simulink model "modelofisicocompleto"  (R2017a)
settings: Solver=VariableStepAuto  StartTime=0.0  StopTime=20  MaxStep=1e-5  RelTol=1e-5
values from neighbouring files (symbols this model uses):
  bcx = 1000    [datoscarro.m]
  bcy = 500    [datoscarro.m]
  Beqtran = (0 + Beqrot/(Rr^2))    (= 27000)    [datoscarro.m]
  Bheqd = (bh  + (beqd/(Rd^2)))    (= 32)    [datoscarro.m]
  bw = 30000    [datoscarro.m]
  g = 9.82    [datoscarro.m]
  Kcy = 1.3e6    (= 1300000)    [datoscarro.m]
  Kw = 1800000    [datoscarro.m]
  lh0 = 10    [datoscarro.m]
  Meq = (mc + Jeq/(Rr^2))    (= 59008)    [datoscarro.m]
  Mheq = (Mh + (Jeqd/(Rd^2)))    (= 48014.2222222)    [datoscarro.m]
  Rd = 0.75    [datoscarro.m]
  Rr = 0.5    [datoscarro.m]
  rt = 15.0    (= 15)    [datoscarro.m]
  rtd = 30    [datoscarro.m]
  xl0 = 5    [datoscarro.m]
  xt0 = xl0    (= 5)    [datoscarro.m]    (also in plot_scene.m = -20)
  yl0 = yt0 - l0    (= 34.9181666667)    [datoscarro.m]
  yt0 = 45    [datoscarro.m]
settings Model: Creator=tomas  LastModifiedBy=tomas

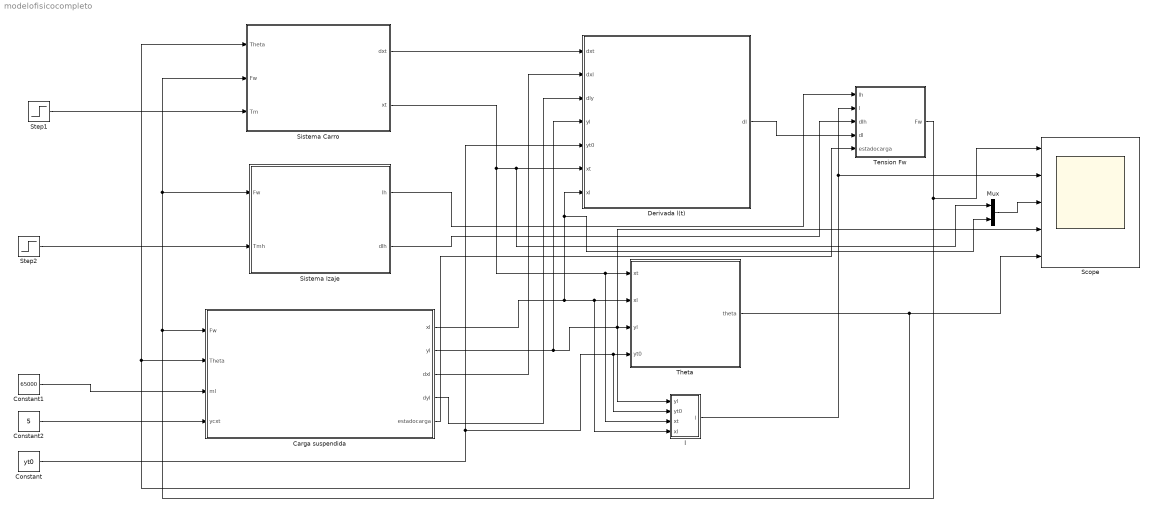
== system modelofisicocompleto ==
  Carga suspendida : Subsystem
  Constant : Constant  Value=yt0
  Constant1 : Constant  Value=65000
  Constant2 : Constant  Value=5
  Derivada l(t) : Subsystem
  Mux : Mux  Inputs=2
  Scope : Scope  NumInputPorts=5
  Sistema Carro : Subsystem
  Sistema Izaje : Subsystem
  Step1 : Step  Time=0  After=1000  SampleTime=0
  Step2 : Step  Time=0  After=25000  SampleTime=0
  Tension Fw : Subsystem
  Theta : Subsystem
  l : Subsystem
  wires:
  Step1/1 -> Sistema Carro/3(Tm)
  Sistema Carro/2(xt) -> l/3(xt), Theta/1(xt), Mux/1, Derivada l(t)/6(xt)
  Sistema Carro/1("dxt ") -> Derivada l(t)/1(dxt)
  Sistema Izaje/1(lh) -> Tension Fw/1(lh)
  Sistema Izaje/2(dlh) -> Tension Fw/3(dlh)
  Carga suspendida/1(xl) -> Mux/2, Derivada l(t)/7(xl), l/4(xl), Theta/2(xl)
  Carga suspendida/2(yl) -> l/1(yl), Theta/3(yl), Scope/4, Derivada l(t)/4(yl)
  Carga suspendida/3(dxl) -> Derivada l(t)/2(dxl)
  Carga suspendida/4(dyl) -> Derivada l(t)/3(dly)
  Derivada l(t)/1(dl) -> Tension Fw/4(dl)
  Constant/1 -> l/2(yt0), Theta/4(yt0), Derivada l(t)/5(yt0)
  l/1("l ") -> Scope/2, Tension Fw/2(l)
  Tension Fw/1("Fw ") -> Sistema Carro/2(Fw), Sistema Izaje/1(Fw), Carga suspendida/1(Fw), Scope/1
  Constant1/1 -> Carga suspendida/3(ml)
  Constant2/1 -> Carga suspendida/4(ycxt)
  Carga suspendida/5("estadocarga ") -> Tension Fw/5(estadocarga)
  Mux/1 -> Scope/3
  Step2/1 -> Sistema Izaje/2(Tmh)
  Theta/1("theta ") -> Scope/5, Sistema Carro/1(Theta), Carga suspendida/2(Theta)

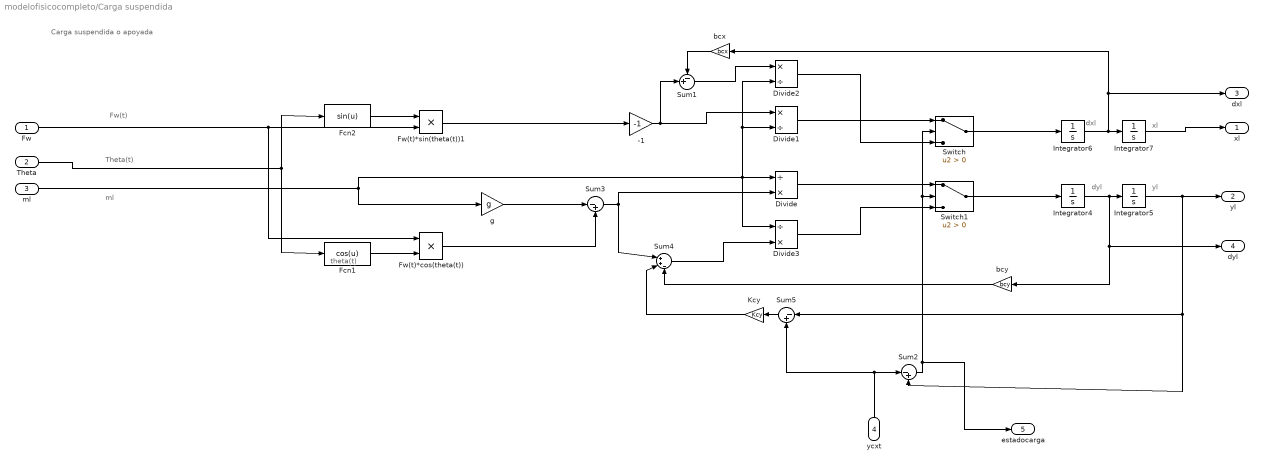
== system modelofisicocompleto/Carga suspendida ==
  note: Carga suspendida o apoyada
  note: Theta(t)
  note: Fw(t)
  note: ml
  note: theta(t)
  note: dyl
  note: yl
  note: dxl
  note: xl
  Fw : Inport
  Theta : Inport  Port=2
  ml : Inport  Port=3
  ycxt : Inport  Port=4
  -1 : Gain  Gain=-1
  Divide : Product  Inputs=/*
  Divide1 : Product  Inputs=*/
  Divide2 : Product  Inputs=*/
  Divide3 : Product  Inputs=/*
  Fcn1 : Fcn  Expr=cos(u)
  Fcn2 : Fcn  Expr=sin(u)
  Fw(t)*cos(theta(t)) : Product
  Fw(t)*sin(theta(t))1 : Product
  Integrator4 : Integrator
  Integrator5 : Integrator  InitialCondition=yl0
  Integrator6 : Integrator
  Integrator7 : Integrator  InitialCondition=xl0
  Kcy : Gain  Gain=Kcy
  Sum1 : Sum  Inputs=-+|
  Sum2 : Sum  Inputs=|-+
  Sum3 : Sum  Inputs=|-+
  Sum4 : Sum  Inputs=|++-
  Sum5 : Sum  Inputs=|-+
  Switch : Switch  Criteria=u2 > Threshold
  Switch1 : Switch  Criteria=u2 > Threshold
  bcx : Gain  Gain=bcx
  bcy : Gain  Gain=bcy
  g : Gain  Gain=g
  xl : Outport
  yl : Outport  Port=2
  dxl : Outport  Port=3
  dyl : Outport  Port=4
  "estadocarga " : Outport  Port=5
  wires:
  Fcn2/1 -> Fw(t)*sin(theta(t))1/1
  Theta/1 -> Fcn1/1, Fcn2/1
  g/1 -> Sum3/1
  Fcn1/1 -> Fw(t)*cos(theta(t))/2
  Fw(t)*cos(theta(t))/1 -> Sum3/2
  Fw/1 -> Fw(t)*cos(theta(t))/1, Fw(t)*sin(theta(t))1/2
  ml/1 -> g/1, Divide1/2, Divide2/2, Divide3/1, Divide/1
  Integrator7/1 -> xl/1
  Integrator6/1 -> bcx/1, dxl/1, Integrator7/1
  Fw(t)*sin(theta(t))1/1 -> -1/1
  Integrator5/1 -> Sum2/2, Sum5/1, yl/1
  Divide1/1 -> Switch/1
  -1/1 -> Sum1/2, Divide1/1
  Integrator4/1 -> dyl/1, bcy/1, Integrator5/1
  Sum3/1 -> Sum4/1, Divide/2
  Switch/1 -> Integrator6/1
  bcx/1 -> Sum1/1
  Sum2/1 -> "estadocarga "/1, Switch1/2, Switch/2
  ycxt/1 -> Sum2/1, Sum5/2
  Sum1/1 -> Divide2/1
  Divide2/1 -> Switch/3
  Sum4/1 -> Divide3/2
  Divide3/1 -> Switch1/3
  Switch1/1 -> Integrator4/1
  Divide/1 -> Switch1/1
  Sum5/1 -> Kcy/1
  Kcy/1 -> Sum4/2
  bcy/1 -> Sum4/3

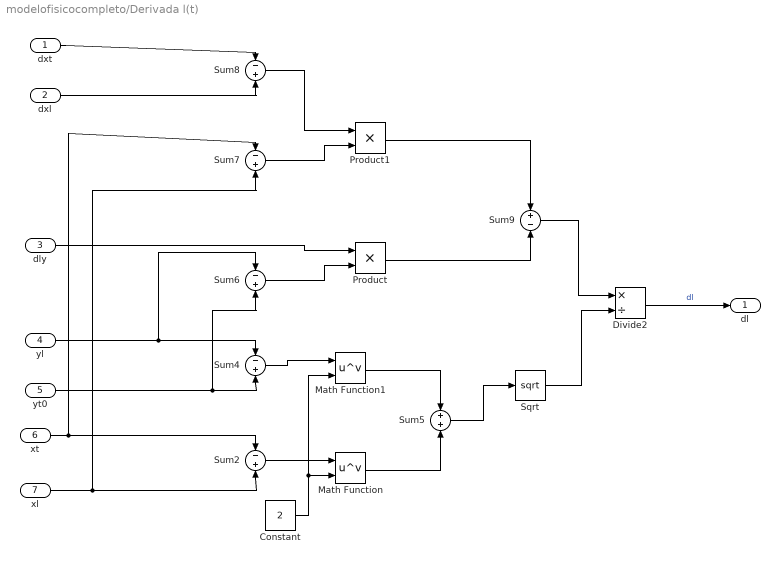
== system modelofisicocompleto/Derivada l(t) ==
  dxt : Inport
  dxl : Inport  Port=2
  dly : Inport  Port=3
  yl : Inport  Port=4
  yt0 : Inport  Port=5
  xt : Inport  Port=6
  xl : Inport  Port=7
  Constant : Constant  Value=2
  Divide2 : Product  Inputs=*/
  Math Function : Math  Operator=pow  SaturateOnIntegerOverflow=on
  Math Function1 : Math  Operator=pow  SaturateOnIntegerOverflow=on
  Product : Product
  Product1 : Product
  Sqrt : Sqrt  SaturateOnIntegerOverflow=on
  Sum{2,4,6..8} (5 alike) : Sum  Inputs=-+
  Sum5 : Sum
  Sum9 : Sum  Inputs=+-
  dl : Outport
  wires:
  Divide2/1 -> dl/1  "dl"
  dly/1 -> Product/1
  yl/1 -> Sum6/1, Sum4/1
  xl/1 -> Sum7/2, Sum2/2
  Product/1 -> Sum9/2
  dxt/1 -> Sum8/1
  Sum5/1 -> Sqrt/1
  Constant/1 -> Math Function1/2, Math Function/2
  yt0/1 -> Sum4/2, Sum6/2
  dxl/1 -> Sum8/2
  Math Function1/1 -> Sum5/1
  Sum8/1 -> Product1/1
  Sum9/1 -> Divide2/1
  Math Function/1 -> Sum5/2
  xt/1 -> Sum7/1, Sum2/1
  Sum6/1 -> Product/2
  Sum7/1 -> Product1/2
  Product1/1 -> Sum9/1
  Sum4/1 -> Math Function1/1
  Sqrt/1 -> Divide2/2
  Sum2/1 -> Math Function/1

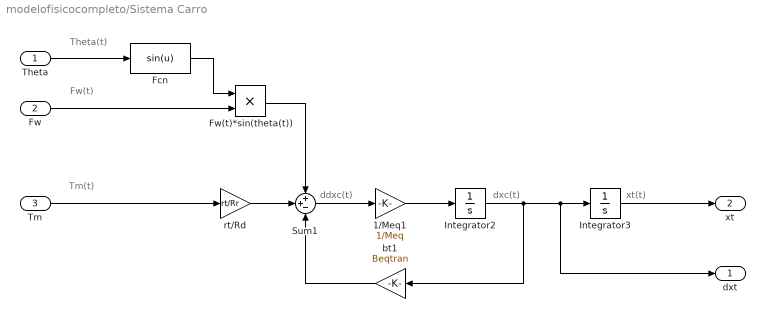
== system modelofisicocompleto/Sistema Carro ==
  note: dxc(t)
  note: xt(t)
  note: ddxc(t)
  note: Theta(t)
  note: Fw(t)
  note: Tm(t)
  Theta : Inport
  Fw : Inport  Port=2
  Tm : Inport  Port=3
  1/Meq1 : Gain  Gain=1/Meq
  Fcn : Fcn  Expr=sin(u)
  Fw(t)*sin(theta(t)) : Product
  Integrator2 : Integrator
  Integrator3 : Integrator  InitialCondition=xt0
  Sum1 : Sum  Inputs=++-
  bt1 : Gain  Gain=Beqtran
  rt/Rd : Gain  Gain=rt/Rr
  "dxt " : Outport
  xt : Outport  Port=2
  wires:
  Integrator3/1 -> xt/1
  Sum1/1 -> 1/Meq1/1
  Fw/1 -> Fw(t)*sin(theta(t))/2
  Fcn/1 -> Fw(t)*sin(theta(t))/1
  rt/Rd/1 -> Sum1/2
  Theta/1 -> Fcn/1
  Fw(t)*sin(theta(t))/1 -> Sum1/1
  1/Meq1/1 -> Integrator2/1
  Tm/1 -> rt/Rd/1
  bt1/1 -> Sum1/3
  Integrator2/1 -> bt1/1, "dxt "/1, Integrator3/1

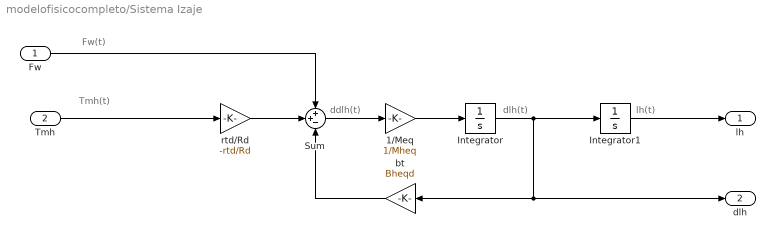
== system modelofisicocompleto/Sistema Izaje ==
  note: lh(t)
  note: dlh(t)
  note: ddlh(t)
  note: Tmh(t)
  note: Fw(t)
  Fw : Inport
  Tmh : Inport  Port=2
  1/Meq : Gain  Gain=1/Mheq
  Integrator : Integrator
  Integrator1 : Integrator  InitialCondition=lh0
  Sum : Sum  Inputs=++-
  bt : Gain  Gain=Bheqd
  rtd/Rd : Gain  Gain=-rtd/Rd
  lh : Outport
  dlh : Outport  Port=2
  wires:
  Integrator/1 -> dlh/1, bt/1, Integrator1/1
  Integrator1/1 -> lh/1
  rtd/Rd/1 -> Sum/2
  bt/1 -> Sum/3
  Fw/1 -> Sum/1
  Tmh/1 -> rtd/Rd/1
  1/Meq/1 -> Integrator/1
  Sum/1 -> 1/Meq/1

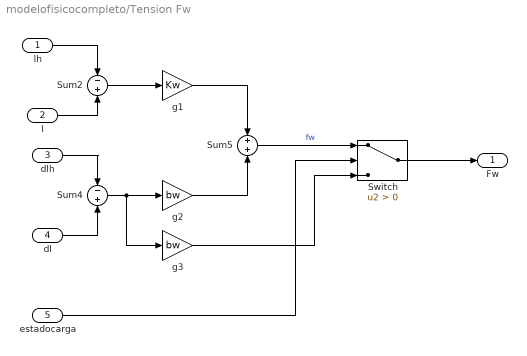
== system modelofisicocompleto/Tension Fw ==
  lh : Inport
  l : Inport  Port=2
  dlh : Inport  Port=3
  dl : Inport  Port=4
  estadocarga : Inport  Port=5
  Sum2 : Sum  Inputs=-+
  Sum4 : Sum  Inputs=-+
  Sum5 : Sum
  Switch : Switch  Criteria=u2 > Threshold
  g1 : Gain  Gain=Kw
  g2 : Gain  Gain=bw
  g3 : Gain  Gain=bw
  "Fw " : Outport
  wires:
  l/1 -> Sum2/2
  lh/1 -> Sum2/1
  dl/1 -> Sum4/2
  g2/1 -> Sum5/2
  Sum5/1 -> Switch/1  "fw"
  Sum4/1 -> g3/1, g2/1
  g1/1 -> Sum5/1
  dlh/1 -> Sum4/1
  Sum2/1 -> g1/1
  Switch/1 -> "Fw "/1
  estadocarga/1 -> Switch/2
  g3/1 -> Switch/3

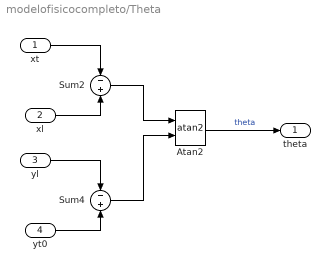
== system modelofisicocompleto/Theta ==
  xt : Inport
  xl : Inport  Port=2
  yl : Inport  Port=3
  yt0 : Inport  Port=4
  Atan2 : Trigonometry  Operator=atan2
  Sum2 : Sum  Inputs=-+
  Sum4 : Sum  Inputs=-+
  "theta " : Outport
  wires:
  Sum4/1 -> Atan2/2
  xt/1 -> Sum2/1
  xl/1 -> Sum2/2
  yt0/1 -> Sum4/2
  Atan2/1 -> "theta "/1  "theta"
  yl/1 -> Sum4/1
  Sum2/1 -> Atan2/1

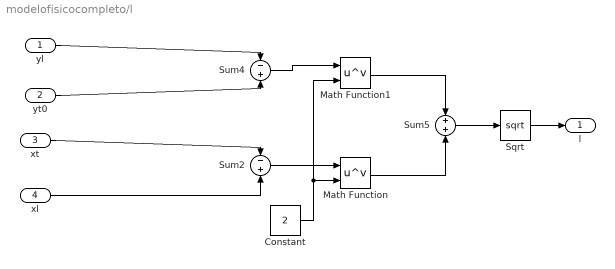
== system modelofisicocompleto/l ==
  yl : Inport
  yt0 : Inport  Port=2
  xt : Inport  Port=3
  xl : Inport  Port=4
  Constant : Constant  Value=2
  Math Function : Math  Operator=pow  SaturateOnIntegerOverflow=on
  Math Function1 : Math  Operator=pow  SaturateOnIntegerOverflow=on
  Sqrt : Sqrt  SaturateOnIntegerOverflow=on
  Sum2 : Sum  Inputs=-+
  Sum4 : Sum  Inputs=-+
  Sum5 : Sum
  "l " : Outport
  wires:
  Sum4/1 -> Math Function1/1
  Sum5/1 -> Sqrt/1
  xt/1 -> Sum2/1
  Math Function1/1 -> Sum5/1
  Math Function/1 -> Sum5/2
  Sqrt/1 -> "l "/1
  Sum2/1 -> Math Function/1
  yl/1 -> Sum4/1
  xl/1 -> Sum2/2
  Constant/1 -> Math Function1/2, Math Function/2
  yt0/1 -> Sum4/2
